simulink library "Sensors"  (R2024a)
settings: Solver=VariableStepAuto  StartTime=0.0  StopTime=10.0  RelTol=1e-3
undefined symbols (not defined in the file): Earth, H0, IMU_Freq, SJK_airport, SJK_direction, WGS84
libraries: sensorgpslib x1, aerolibtransform2 x1, aerolibnav x1, aerolibasang x1
settings Model: Creator=igmso  LastModifiedBy=igmso

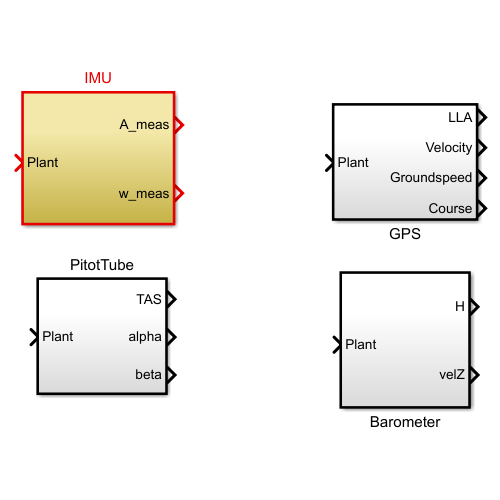
[thumbnail: Simulink's stored preview of the top-level diagram]
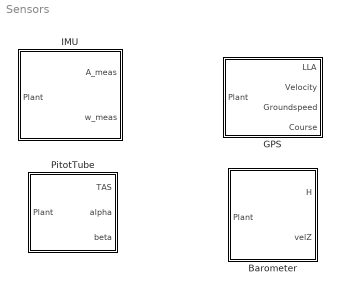
== system Sensors ==
  Barometer : Subsystem  TreatAsAtomicUnit=on  SystemSampleTime=1/400
  GPS : Subsystem  TreatAsAtomicUnit=on  SystemSampleTime=1/10
  IMU : Subsystem  TreatAsAtomicUnit=on
  PitotTube : Subsystem  TreatAsAtomicUnit=on  SystemSampleTime=1/400

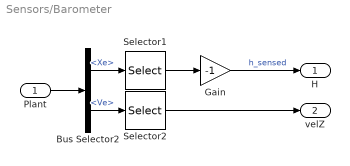
== system Sensors/Barometer ==
  Plant : Inport  SampleTime=1/400
  Bus Selector2 : BusSelector  OutputSignals=Xe,Ve
  Gain : Gain  Gain=-1
  Selector1 : Selector  InputPortWidth=3  IndexOptions=Index vector (dialog)  Indices=3  OutputSizes=1
  Selector2 : Selector  InputPortWidth=3  IndexOptions=Index vector (dialog)  Indices=3  OutputSizes=1
  H : Outport  SampleTime=1/400
  velZ : Outport  Port=2  SampleTime=1/400
  wires:
  Bus Selector2/2 -> Selector2/1  "<Ve>"
  Gain/1 -> H/1  "h_sensed"
  Selector2/1 -> velZ/1
  Bus Selector2/1 -> Selector1/1  "<Xe>"
  Plant/1 -> Bus Selector2/1
  Selector1/1 -> Gain/1

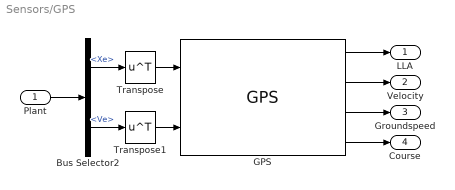
== system Sensors/GPS ==
  Plant : Inport
  Bus Selector2 : BusSelector  OutputSignals=Xe,Ve
  GPS : sensorgpslib/GPS  DispRefFrame=NED  PositionInputFormat=Local  ReferenceLocation=[SJK_airport;SJK_direction]  HorizontalPositionAccuracy=0.025  VerticalPositionAccuracy=0.015  VelocityAccuracy=0.1  DecayFactor=0.999  SeedDouble=67  SimulateUsing=Interpreted execution
      settings: LibrarySourceBlock=mspsensorlib/GPS
  Transpose : Math  Operator=transpose
  Transpose1 : Math  Operator=transpose
  LLA : Outport
  Velocity : Outport  Port=2
  Groundspeed : Outport  Port=3
  Course : Outport  Port=4
  wires:
  Transpose1/1 -> GPS/2
  Transpose/1 -> GPS/1
  Bus Selector2/1 -> Transpose/1  "<Xe>"
  Bus Selector2/2 -> Transpose1/1  "<Ve>"
  GPS/1 -> LLA/1
  GPS/2 -> Velocity/1
  GPS/4 -> Course/1
  Plant/1 -> Bus Selector2/1
  GPS/3 -> Groundspeed/1

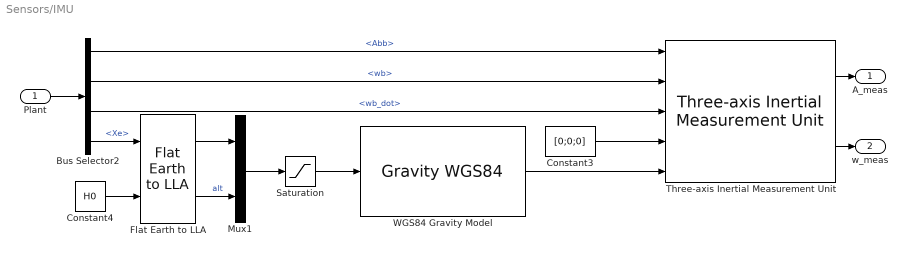
== system Sensors/IMU ==
  Plant : Inport  SampleTime=1/IMU_Freq
  Bus Selector2 : BusSelector  OutputSignals=Abb,wb,wb_dot,Xe
  Constant3 : Constant  Value=[0;0;0]  SampleTime=1/IMU_Freq
  Constant4 : Constant  Value=H0  SampleTime=1/IMU_Freq
  Flat Earth to LLA : aerolibtransform2/Flat Earth to LLA  units=Metric (MKS)  ptype=Earth (WGS84)  F=1/298.257223563  R=6378137  refPosPort=off  LL0=SJK_airport  psi=SJK_direction
  Mux1 : Mux  Inputs=2
  Saturation : Saturate  UpperLimit=2033  LowerLimit=0
  Three-axis Inertial Measurement Unit : aerolibnav/Three-axis Inertial Measurement Unit  units=Metric (MKS)  imu=[0 0 0]  i_Ts=1/800  dtype_a=on  w_a=190  z_a=0.707  a_sf_cc=[1 0 0; 0 1 0; 0 0 1]  a_bias=[0 0 0]  a_sat="[-inf  -inf  -inf  inf inf inf]"  dtype_g=on  w_g=190  z_g=0.707  g_sf_cc=[1 0 0; 0 1 0; 0 0 1]  g_bias=[0 0 0]  g_sens=[0 0 0]  g_sat="[-inf  -inf  -inf  inf inf inf]"  i_rand=on  i_seeds=[23093 23094 23095 23096 23097 23098]  i_pow=[0.00001 0.00001 0.00001 0.000001 0.000001 0.000001]
  "WGS84 Gravity Model  " : GravityWGS84
  A_meas : Outport  SampleTime=1/IMU_Freq
  w_meas : Outport  Port=2  SampleTime=1/IMU_Freq
  wires:
  Saturation/1 -> "WGS84 Gravity Model  "/1
  Three-axis Inertial Measurement Unit/1 -> A_meas/1
  Three-axis Inertial Measurement Unit/2 -> w_meas/1
  Flat Earth to LLA/1 -> Mux1/1
  Constant4/1 -> Flat Earth to LLA/2
  Flat Earth to LLA/2 -> Mux1/2  "alt"
  Bus Selector2/1 -> Three-axis Inertial Measurement Unit/1  "<Abb>"
  "WGS84 Gravity Model  "/1 -> Three-axis Inertial Measurement Unit/5
  Bus Selector2/4 -> Flat Earth to LLA/1  "<Xe>"
  Plant/1 -> Bus Selector2/1
  Mux1/1 -> Saturation/1
  Bus Selector2/3 -> Three-axis Inertial Measurement Unit/3  "<wb_dot>"
  Constant3/1 -> Three-axis Inertial Measurement Unit/4
  Bus Selector2/2 -> Three-axis Inertial Measurement Unit/2  "<wb>"

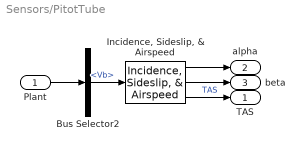
== system Sensors/PitotTube ==
  Plant : Inport  SampleTime=1/400
  Bus Selector2 : BusSelector  OutputSignals=Vb
  "Incidence, Sideslip, & Airspeed" : aerolibasang/Incidence, Sideslip, & Airspeed
  TAS : Outport
  alpha : Outport  Port=2
  beta : Outport  Port=3
  wires:
  "Incidence, Sideslip, & Airspeed"/2 -> beta/1
  "Incidence, Sideslip, & Airspeed"/1 -> alpha/1
  Bus Selector2/1 -> "Incidence, Sideslip, & Airspeed"/1  "<Vb>"
  "Incidence, Sideslip, & Airspeed"/3 -> TAS/1  "TAS"
  Plant/1 -> Bus Selector2/1
